simulink model "interval_of_fonem"  (R2017b)
settings: Solver=FixedStepDiscrete  StartTime=0.0  StopTime=13.4037  RelTol=1e-3
PreLoadFcn:
  | function a = fcn1111(u)
  | number = zeros(10,1);
  | move   = zeros(10,1);
  | 
  | a = struct('numbers',number,'movement', move);
  | 
  | busInfo = Simulink.Bus.createObject(a);
  | end
values from neighbouring files (symbols this model uses):
  choseFilter = [1 2 3 4 5 6 7 8 9 10 11 12 13 14 15 16 17]    [SetParam.m]
  conF = zeros(1,diff,'double')    [SetParam.m]
  Fh = 44100    [SetParam.m]
  Fl = 20    [SetParam.m]
  Fs = 44100    [SetParam.m]
  NFilt = 20    [SetParam.m]
  samplesize = 2048    [SetParam.m]
undefined symbols (not defined in the file or in its folder): get
libraries: dspsnks4 x2, dspvision x1, dspobslib x1
settings Model: Creator=root  LastModifiedBy=root

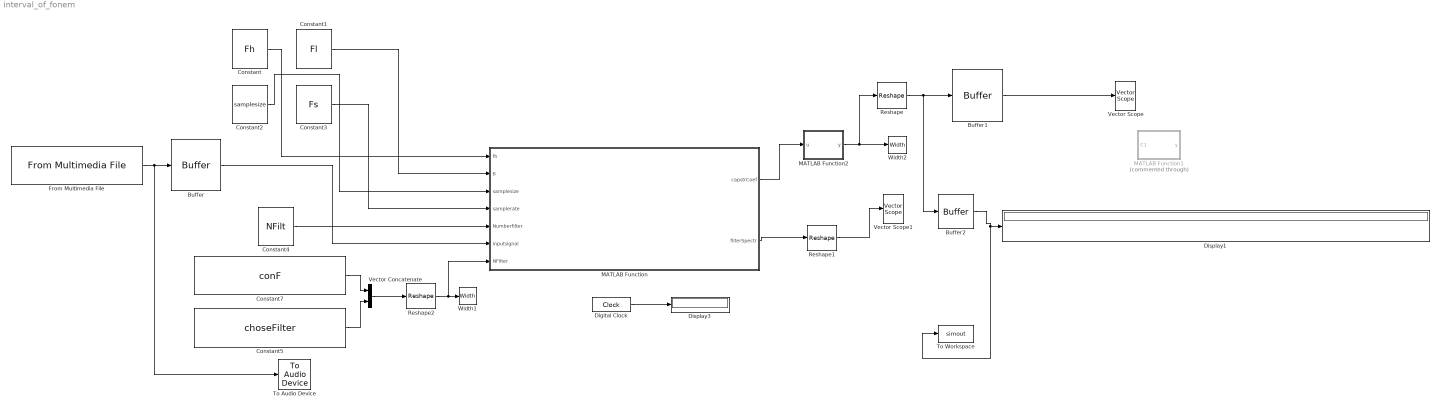
== system interval_of_fonem ==
  Buffer : Buffer  N=2048  V=1024  OutputFrames=off
  Buffer1 : Buffer  N=20  OutputFrames=off
  Buffer2 : Buffer  N=20  OutputFrames=off
  Constant : Constant  Value=Fh
  Constant1 : Constant  Value=Fl
  Constant2 : Constant  Value=samplesize
  Constant3 : Constant  Value=Fs
  Constant4 : Constant  Value=NFilt
  Constant5 : Constant  Value=choseFilter  OutDataTypeStr=double
  Constant7 : Constant  Value=conF  OutDataTypeStr=double
  Digital Clock : DigitalClock  SampleTime=1/Fs
  Display1 : Display
  Display3 : Display
  From Multimedia File : dspvision/From Multimedia File  inputFilename=/home/stark/git/AudioFilter/AudioAnalizer/OriginalSignal/01-01-01-_AudioTrimmer_com_1_.wav  loop=on  numPlays=inf  outputStreams=Audio only  videoDataType=single  audioDataType=double  inheritSampleTime=on  userDefinedSampleTime=1/30  noAudioOutput=off  isIntensityVideo=off  fourcc=RGB  colorVideoFormat=Separate color signals  outputEOF=off  dataOrg=Column-major  audioFrameSize=2048  computeAudioFrameSize=off  outSamplingMode=Frame based
      settings: SourceProductBaseCode=VP
  MATLAB Function : MATLAB Function  TreatAsAtomicUnit=on
  MATLAB Function1 : MATLAB Function  Commented=through  TreatAsAtomicUnit=on
  MATLAB Function2 : MATLAB Function  TreatAsAtomicUnit=on
  Reshape : Reshape
  Reshape1 : Reshape
  Reshape2 : Reshape
  To Audio Device : dspobslib/To Audio Device  deviceName=Default  inheritSampleRate=on  sampleRate=44100  deviceDatatype=Determine from input data type  autoBufferSize=on  bufferSize=4096  queueDuration=1.0  defaultOutputChannelMapping=on  outputChannelMapping=1:2  outputNumUnderrunSamples=off
      settings: SourceProductName=DSP System Toolbox  SourceProductBaseCode=DS
  To Workspace : ToWorkspace  VariableName=simout  SampleTime=-1
      settings: Save2DSignal=2-D array (concatenate along first dimension)
  Vector Concatenate : Concatenate
  Vector Scope : dspsnks4/Vector Scope  ScopeProperties=on  Domain=Time  HorizSpan=1  DisplayProperties=off  AxisGrid=on  Memory=off  FrameNumber=on  AxisLegend=off  AxisZoom=off  OpenScopeAtSimStart=on  OpenScopeImmediately=off  FigPos=get(0,'defaultfigureposition')  AxisProperties=off  XUnits=Hertz  XRange=[0...Fs/2]  InheritXIncr=on  XIncr=1  XLabel=Time  XLimit=Auto  XMin=0  XMax=1  XStart=0  YUnits=dB  YLabel=Amplitude  LineProperties=off  XAxisParamsVer=6.9
      settings: SourceProductName=DSP System Toolbox  SourceProductBaseCode=DS  YMin=-70  YMax=70
  Vector Scope1 : dspsnks4/Vector Scope  ScopeProperties=on  Domain=Time  HorizSpan=1  DisplayProperties=off  AxisGrid=on  Memory=off  FrameNumber=on  AxisLegend=off  AxisZoom=off  OpenScopeAtSimStart=on  OpenScopeImmediately=off  FigPos=get(0,'defaultfigureposition')  AxisProperties=off  XUnits=Hertz  XRange=[0...Fs/2]  InheritXIncr=on  XIncr=1  XLabel=Time  XLimit=Auto  XMin=0  XMax=1  XStart=0  YUnits=dB  YLabel=Amplitude  LineProperties=off  XAxisParamsVer=6.9
      settings: SourceProductName=DSP System Toolbox  SourceProductBaseCode=DS  YMin=-1  YMax=1
  Width1 : Width
  Width2 : Width
  wires:
  From Multimedia File/1 -> To Audio Device/1, Buffer/1
  Constant/1 -> MATLAB Function/1(fh)
  Constant1/1 -> MATLAB Function/2(fl)
  Constant2/1 -> MATLAB Function/3(samplesize)
  Constant3/1 -> MATLAB Function/4(samplerate)
  Buffer/1 -> MATLAB Function/6(inputsignal)
  MATLAB Function/1(capstrCoef) -> MATLAB Function2/1(u)
  MATLAB Function2/1(y) -> Width2/1, Reshape/1
  Buffer1/1 -> Vector Scope/1
  Reshape/1 -> Buffer2/1, Buffer1/1
  MATLAB Function/2(filterSpectr) -> Reshape1/1
  Reshape1/1 -> Vector Scope1/1
  Vector Concatenate/1 -> Reshape2/1
  Constant4/1 -> MATLAB Function/5(Numberfilter)
  Constant7/1 -> Vector Concatenate/1
  Constant5/1 -> Vector Concatenate/2
  Reshape2/1 -> Width1/1, MATLAB Function/7(NFilter)
  Digital Clock/1 -> Display3/1
  Buffer2/1 -> To Workspace/1, Display1/1

== matlab function interval_of_fonem/MATLAB Function1 ==
  data: C1 input; y output
function y = lengthFonem(C1)
%берем первые десять коеффицыентов
C1=C1(:,2:14);
%рассчитаем коеффицыент регресии
I=3;%соседние отчеты
rsum=-3:1:3;
rsum=sum(rsum.^2);
res_N=0;
ri=[];

%щитаем сумму отчетов в окрестности
% C11=C1(1:7,1);
n=1; 
% endi=length(C1(:,1));
endi=length(C1(:,1));
start=4;
i=1;
newN=1;
median=I+I+1;
n=1:1:16;
regressC=zeros(1,13,'double');
regC=[];
coder.extrinsic('cat');
i=1;
    %хитрое окно
%     for filtCentre=1:1:length(C1(:,1))
        filtCentre=1;
      if filtCentre<=I
        %начинаем окно
        if   filtCentre == 1
            regC=C1(filtCentre,i)*0+C1(filtCentre+1,i)*1+C1(filtCentre+2,i)*2+C1(filtCentre+3,i)*3;
            regressC(filtCentre,i)=regC;
            filtCentre=filtCentre+1;
        end
        
        
         if   filtCentre == 2
             regC=C1(filtCentre-1,i)*(-1)+C1(filtCentre,i)*(0)+C1(filtCentre+1,i)*1+...
             C1(filtCentre+2,i)*2+C1(filtCentre+3,i)*3;
            regressC(filtCentre,i)=regC*5;
            filtCentre=filtCentre+1;
         end
       
        if   filtCentre == I
            regC=C1(filtCentre-2,i)*(-2)+C1(filtCentre-1,i)*(-1)+C1(filtCentre,i)*0+...
            C1(filtCentre+1,i)*1+C1(filtCentre+2,i)*2+C1(filtCentre+3,i)*3;
            regressC(filtCentre,i)=regC*6;
            filtCentre=filtCentre+1;
        end
      end
  
     %окно в идеальных условиях
       for filtCentre=I+1:1:length(C1(:,1))-I
                 regC=[];
                for i11=-I:1:I
                    indC1=C1(filtCentre + i11,i)*i11;
                    regC = cat (1, regC , indC1);
%                     regC=[regC C1(filtCentre + i11,i)*i11];

                end
                regressC(filtCentre,i)=sum(regC);
                I=3;
                regC=[];      
      end 
%       filtCentre=filtCentre+1;
       
   if endi-filtCentre <= I
               %завершаем окно
         if   endi-filtCentre == I
            regC=C1(filtCentre+1,i)*(1)+C1(filtCentre+2,i)*(2)+C1(filtCentre,i)*0 +...
            C1(filtCentre-1,i)*(-1)+C1(filtCentre-2,i)*(-2)+C1(filtCentre-3,i)*(-3); 
            filtCentre=filtCentre+1;
            regressC(filtCentre,i)=regC;
         
         end
         
         if   endi-filtCentre == 2
             regC=C1(filtCentre+1,i)*1+C1(filtCentre,i)*0+C1(filtCentre-1,i)*(-1)+...
             C1(filtCentre-2,i)*(-2)+C1(filtCentre-3,i)*(-3);
          filtCentre=filtCentre+1;
            regressC(filtCentre,i)=regC;
            
           
         end
      
        if   endi-filtCentre == 1
            regC=C1(filtCentre,i)*0+C1(filtCentre-1,i)*(-1)+C1(filtCentre-2,i)*(-2)+C1(filtCentre-3,i)*(-3);
            filtCentre=filtCentre+1;
            regressC(filtCentre,i)=regC;
            
        end
     
   end   
       
    
    for n=1:1:16
    regressC(n,:)=regressC(n,:)./rsum;
    end

N=length(C1(1,:));
 for n=1:1:length(C1(:,1))%-3
    
%         
%         S(n)=sum(NEww(n,:))./N;
       S(n)=sum(regressC(n,:))./N;
    
end





y = S;

== matlab function interval_of_fonem/MATLAB Function ==
  data: fh input double; capstrCoef output double size=[1,20] [0..20]; fl input double; samplesize input double; samplerate input double; Numberfilter input double; inputsignal input double size=[2048,1] [0..2048]; filterSpectr output size=[1,1025] [0..1025]; NFilter input double size=[1 20]
function [capstrCoef,filterSpectr]= melCapstr(fh,fl,samplesize,samplerate,Numberfilter,inputsignal,NFilter)
% this function returns the mel-capstr coefficients for each sample in the signal
% signal has length, it contains vectors = length (sample size)
% of the sample size, we have to shield knowing the sampling rate and the period that we need
% for example:
%Fs=44100; we need length sample = 25 - 30ms
%floor(Fs*length sample)=sampleSize;
%floor(44100*25*10^-3)~=1128
%in my case I chose 50ms (2048)
%==========================================================================

Fs=samplerate;
% sampleSize=1128;
sampleSize=samplesize;
coder.extrinsic('hamming');
coder.extrinsic('dct');
hammingWindow=zeros(2048,1,'double');
hammingWindow = hamming(2048,'symmetric');
hammingWindow = hammingWindow';
nMelFilt=Numberfilter;% quantity filters for MFCC analizing
ctrlPointFilt=nMelFilt+2;% quantity points for mel filters
inputSignal=zeros(2048,1,'double');
inputSignal=inputsignal;
a=1;
%===================== discrete fourier transform for each sample in audio signal
startSemple=1;
endSemple=sampleSize;
arrayOfPlots=zeros(576,2048,'double');
vector=zeros(2048,1,'double');
vector=inputSignal;
stepen=sampleSize;
vector1=zeros(1,2048,'double');
[m n]=size(vector);
if m > n
vector1=vector';
end

    new_wector=zeros(1,2048,'double');
    new_wector = vector1;
   

 new_wector=new_wector.*hammingWindow;
 res_val=zeros(1,1025,'double');
L = 2048;             % Length of signal (длина одной выборки для преобразования)
Y = fft(new_wector);%преобразование фурье
P2 = abs(Y/L);%,берем АЧХ и нормируем
P1 = P2(1:L/2+1);% Реальная часть спектра
P1(2:end-1) = 2*P1(2:end-1); % умножаем все на 2 кроме первой постоянной составляющей
res_val=P1;
f = Fs*(0:(L/2))/L;%массив частот


%++++++++++++++++++++++++++++++++++++++++++++++++++++++++++++++++++++++++++
%friquency to mel
fmelL=1127*log(1 + (fl / 700) );
fmelH=1127*log(1 + (fh / 700) );
n=(fmelH-fmelL)/(nMelFilt+1);%20 filters, 22 fixed point for filters
FMel=fmelL:n:fmelH; 
%+++++++++++++++++++++++++++++++++++++++++++++++++++++++++++++++++++++++++++
h=zeros(1,ctrlPointFilt,'double');
shag=zeros(1,ctrlPointFilt,'double');
%mel to friquency
     for k=1:1:ctrlPointFilt

        h(k)=700*((exp(FMel(k)/1127))-1);

    end

%point for mel filter
    for i=1:1:ctrlPointFilt
         
        shag(i) = floor(((1025 + 1) * h(i)) / 44100);
    
    end

%++++++++++++++++++++++++++++++++++++++++++++++++++++++++++++++++++++++++++
%create mel filterbank
k=1;
fbank=zeros(nMelFilt,floor((2048/2)+1));
for i=2:1:nMelFilt+1
    f_m_minus = shag(i - 1);
     f_m = shag(i);
      f_m_plus = shag(i + 1);
      
          for k=1+f_m_minus:f_m

          fbank(i - 1, k) = (k - shag(i - 1)) / (shag(i) - shag(i - 1));

          end

          for k=1+f_m:f_m_plus

           fbank(i - 1, k) = (shag(i + 1) - k) / (shag(i + 1) - shag(i));

          end
end
%++++++++++++++++++++++++++++++++++++++++++++++++++++++++++++++++++++++++++
    
    mel=zeros(1,nMelFilt);
    Mel_coef=zeros(20,1025,'double');
    filterSpectr1=zeros(20,1025,'double');
% =========================================================================
%array for chose filter and show it's spectr in summary array
priznakArr=zeros(1,nMelFilt,'double');
filterFlag=NFilter;
[m n]=size(filterFlag);
% n=SizeN;
if n==nMelFilt
priznakArr=filterFlag;
end

if n==1
    B=zeros(1,nMelFilt);
    B(n)=n;
    ind=B(n);
end
if n > 1 && n~=nMelFilt
    B = sort(filterFlag);
    A = zeros(1,nMelFilt-n,'double');
    B = cat(2,B,A);
    priznakArr=zeros(1,length(B),'double');
    for i=1:1:nMelFilt
        N=B(i);
        if N > 0
            priznakArr(N)=N;
        
        end
    end
end
%=========================================================================
%hier make summary array for spectr triangular filters
fbank1=zeros(20,1025,'double');
fbank1=fbank;
UniArr=zeros(1,1025,'double');
      g=1;
    mel=zeros(1,nMelFilt);
    
     for i=1:nMelFilt
         if priznakArr(i)>0
            Mel_coef(i,:)=res_val(1,:).*fbank1(i,:);
            mel(i)= sum(Mel_coef(i,:));
            mel(i)=log(mel(i));
         else
            Mel_coef(i,:)=res_val(1,:).*0;
            mel(i)= sum(Mel_coef(i,:));
            mel(i)=log(mel(i));
         end
     end
     
     for i=1:1:20
       for  j=1:1:1025
         
             if Mel_coef(i,j) > 0 || Mel_coef(i,j) < 0 
                 UniArr(j)=Mel_coef(i,j);

             end
       end
       
     end
%      Ui=zeros(1,1025,'double');
     filterSpectr = UniArr./max(UniArr);
     
%==========================================================================
%mel coefficients
    g=1;
    mel=zeros(1,nMelFilt);
%     while g<=length(res_val(:,1))
      
     for i=1:nMelFilt
            Mel_coef(i,:)=(res_val(g,:).^2).*fbank(i,:);
            mel(i)= sum(Mel_coef(i,:));
            mel(i)=log(mel(i));
    end
%            
%         gg(g,:)=mel; 
%     g=g+1;      
    
%     end  
%==========================================================================
%getting mel-capstr coefficients using discrete cosinus tranform
C=zeros(1,20,'double');
C1=zeros(1,20,'double');
% for n=1:1:nMelFilt
%         for m=1:1:nMelFilt
% 
%             C(m)=mel(m)*cos(((pi*n)*((m+(1/2))))/nMelFilt);
%            
%         end
%         C1(n)=sum(C);
% end
% 
% capstrCoef=zeros(1,20,'double');
% capstrCoef=C1;

%  N=1;
% L=length(mel(:,1));
% ArrA=zeros(1,20,'double');

%         for N=1:1:L
%             ArrA=mel(N,:);
            C1=dct(mel);
%             C1(N,:)= C1(N,:)./max(C1(N,:));
%         end
capstrCoef=zeros(1,20,'double');
capstrCoef=C1;
%==========================================================================
end

== matlab function interval_of_fonem/MATLAB Function2 ==
  data: u input double size=[1,20] [1..20]; y output double size=[1,20] [0..20]
function y = costil(u)
y=zeros(1,20,'double');
            u=u;
            coder.varsize('u', [1 20]); 
%         if length(u)< 585
% 
%             y = u(1:512);
%         end
%             
%         elseif length(u)< 1083
%             
%             y=zeros(1084,1,'double');
%             
%         end
 y = u(1,1:20);
end

% y = u;
